simulink model "controlMCUSlugsMKII"  (Simulink 6.6)
settings: Solver=FixedStepDiscrete  StartTime=0.0  StopTime=10.0  FixedStep=0.01  RelTol=1e-3
InitFcn:
  | mcuInit
values from neighbouring files (symbols this model uses):
  T = 0.01    [initGPS.m]    (also in mcuInit.m)
undefined symbols (not defined in the file or in its folder): apSampleTime, bankCommandLimit, baseHeight, bda, bde, bdr, bdt, bICda, bICde, bICdr, bICdt, controlMCUInit, daLimit, deLimit, drLimit, dtLimit, getAccBias, getAccels, getAttitude, getMidLevelCommands, getPassValues, getPidIdx, getWP, getXYZ, gsRead, ISA_g, mda, mde, mdr, mdt, mICda, mICde, mICdr, mICdt, pitchCommandLimit, prepareTelemetry, protParseDecode, protParseDecodeGS, readIpc, send2GS, setCurrentCommands, setDiagnosticFloat, setDiagnosticShort, setNavLat, setNavLong, setNavNav, u1, u2, updateEuler, updateLoad, updatePQR, updatePWM, updatePWM2, y1
libraries: dsPICdrivers x82, simulink x43, SLUGS_Library x27, aerolibconvert2 x3, aerolibutil x3
(part 5 of 5)

== matlab function Trim Vals/Bufffer IC/Buffer IC Channel ==
  data: latest input inherited; history output inherited
function history = bufferICValues(latest)
% This block supports an embeddable subset of the MATLAB language.
% See the help menu for details. 

persistent oldValues;

if isempty(oldValues)
    oldValues = uint16([0 0 0 0 0 0 0]);
end

history = uint16([0 0 0 0 0 0 0]);

for i=7:-1:2
    oldValues(i) = oldValues(i-1);
	history(i) = oldValues(i-1);
end
	
oldValues(1) = latest;
history(1) = latest;

== matlab function Inner Loop/ Navigation/Navigation/Compute WP Index/Compute P/Compute T in Frenet/Normalize Vector/Norm/Subsystem3/Embedded MATLAB Function ==
  data: x input inherited; y input inherited; xDoty output inherited
function xDoty = myDot(x,y)
% This block supports an embeddable subset of the MATLAB language.
% See the help menu for details. 

xDoty = x(1)*y(1) + x(2)*y(2) + x(3)*y(3);

== matlab function Trim Vals/Bufffer IC/Buffer IC Channel1 ==
  data: latest input inherited; history output inherited
function history = bufferICValues(latest)
% This block supports an embeddable subset of the MATLAB language.
% See the help menu for details. 

persistent oldValues;

if isempty(oldValues)
    oldValues = uint16([0 0 0 0 0 0 0]);
end

history = uint16([0 0 0 0 0 0 0]);

for i=7:-1:2
    oldValues(i) = oldValues(i-1);
	history(i) = oldValues(i-1);
end
	
oldValues(1) = latest;
history(1) = latest;

== matlab function Inner Loop/ Navigation/Longitudinal Channel/Compute Airspeed/Subsystem1/negprotect ==
  data: val input inherited; zpVal output inherited
function zpVal = negProt(val)
% This block supports an embeddable subset of the MATLAB language.
% See the help menu for details. 

if val >= single(0.001)
    zpVal = val;
else
    zpVal = single(0.001);
end

== matlab function Inner Loop/ Navigation/Navigation/Compute WP Index/Compute P/Get Circles/Compute Circles ==
  data: sd input inherited; O output inherited; cd input inherited; WP1 input inherited; R input inherited; T1 input inherited; P output inherited; Pch output inherited; T2 input inherited; PchB output inherited
function [O,P,Pch, PchB] = getO(sd, cd, WP1, R, T1, T2)
    % This block supports an embeddable subset of the MATLAB language.
    % See the help menu for details.

    % rotate the vector delta degrees
    r_vec = zeros(3,1);
    r_vec(1) = -T1(1)*cd -T1(2)*sd;
    r_vec(2) = T1(1)*sd -T1(2)*cd;

    %compute M
    if localAbs(sd)>0.01
        M = localAbs(R/sd);
    else
        M = single(0);
    end

    %find the distance from WP
    P = M*cd;

    % find the center of the circle
    O = WP1 + r_vec.*M;

    % find the tangent points
    Pch = WP1-T1*P;
    PchB = WP1 + T2*P;
end

function absVal = localAbs(x)
    if x < 0
        absVal = single(-1*x);
    else
        absVal = single(x);
    end
end

== matlab function Inner Loop/ Navigation/Navigation/Compute WP Index/Compute P/Get Circles/Compute CCW Angle From 2 Vectors/Embedded MATLAB Function1 ==
  data: rawAngle input inherited; angle output inherited
function angle = mapToTwoPi(rawAngle)

 if(rawAngle < 0)
  angle = rawAngle + 2*pi;
 else
  angle = rawAngle;   
 end

== matlab function Inner Loop/ Navigation/Navigation/Compute WP Index/Embedded MATLAB Function ==
  data: wpStart input inherited; wpCount input inherited; wp0 output inherited; swIncrement input inherited; wp1 output inherited; wp2 output inherited; wpEnabl input inherited
function [wp0,wp1, wp2] = getNextWP(wpStart, wpCount, swIncrement, wpEnabl)

% Declare static variables
persistent fromWP;
persistent toWP;
persistent totoWP;

%initialize the static variables
if isempty(fromWP)
    fromWP = uint8(wpStart);
    toWP = uint8(fromWP+1);
    % check if there are more than 2 WPs
    if wpCount > toWP + 1
        totoWP = uint8(toWP+1);
    else
        totoWP = uint8(fromWP);
    end
end

%if WP Nav was just enabled
if wpEnabl == 1
    fromWP = uint8(0);
    toWP = uint8(1);
    totoWP = uint8(2);
end;

% if there is a change of wp
if swIncrement == 1
    fromWP = toWP;
    toWP = totoWP;
    totoWP = totoWP +1;
    if (totoWP>wpCount)
        totoWP = wpStart;
    end
end

wp0 = fromWP;
wp1 = toWP;
wp2 = totoWP;

== matlab function Inner Loop/ Navigation/Navigation/Compute WP Index/Embedded MATLAB Function1 ==
  data: swDistanceRdy input inherited; timeLimit input inherited; swIncrement output inherited
function swIncrement  = computeSwitch(swDistanceRdy, timeLimit)

% Declare static variables
persistent oldSw;
persistent internalTimer;

%initialize the static variables
if isempty(oldSw)
    oldSw = uint8(0);
    internalTimer = uint16(0);
    % check if there are more than 2 WPs
end 

swIncrement = 0;

%if we just had a flip
if swDistanceRdy == 1 && oldSw == 0
    % if enough time has passed that another switch is valid
    if internalTimer > timeLimit
        swIncrement = 1;
        internalTimer = uint16(0);
    end
end;

internalTimer = internalTimer +1;
oldSw = swDistanceRdy;

== matlab function Inner Loop/ Navigation/Longitudinal Channel/myMux Fun1 ==
  data: u1 input inherited; y output inherited; u2 input inherited
function y = myMux(u1, u2)
% This block supports an embeddable subset of the MATLAB language.
% See the help menu for details. 

y = [u1(1); u2(1)];

== matlab function Inner Loop/ Navigation/Navigation/Park, Deyst & How Lat Accel Cmd/myMux Fun2 ==
  data: u1 input inherited; y output inherited; u2 input inherited; u3 input inherited
function y = myMux(u1, u2, u3)
% This block supports an embeddable subset of the MATLAB language.
% See the help menu for details. 

y = [u1(1); u2(1); u3(1)];

== matlab function Inner Loop/ Navigation/Longitudinal Channel/0.5 sec  tau for Turns/Embedded MATLAB Function ==
  data: u input inherited; y output inherited; T input inherited; f input inherited
function y = fcn(u,T,f)
% This block supports an embeddable subset of the MATLAB language.
% See the help menu for details. 

persistent a
persistent b
persistent y_km1
persistent u_km1
if isempty(a)
    %tf = [T*omega/(2+T*omega) T*omega/(2+T*omega)],[1 (T*omega-2)/(T*omega+2)]
    %tf = [a a],[1 -b]
    omega = 2*pi*f;
    a=T*omega/(2+T*omega);
    b=-(T*omega-2)/(T*omega+2);
    y_km1=u;
    u_km1=u;
end

y = a*(u+u_km1)+b*y_km1;
y_km1=y;
u_km1=u;

== matlab function Inner Loop/ Navigation/Lateral Channel/Sideslip Compensation/Bank to Psi Dot/negprotect ==
  data: val input inherited; zpVal output inherited
function zpVal = negProt(val)
% This block supports an embeddable subset of the MATLAB language.
% See the help menu for details. 

if val >= single(0.001)
    zpVal = val;
else
    zpVal = single(0.001);
end

== matlab function Inner Loop/ Navigation/Navigation/Park, Deyst & How Lat Accel Cmd/Compute Eta/negprotect ==
  data: val input inherited; zpVal output inherited
function zpVal = negProt(val)
% This block supports an embeddable subset of the MATLAB language.
% See the help menu for details. 

if val >= single(0.001)
    zpVal = val;
else
    zpVal = single(0.001);
end

== matlab function Inner Loop/ Navigation/Navigation/Park, Deyst & How Lat Accel Cmd/GainSchedule L2 and Get Groundspeed/Norm /Square Vx and Vy Only. Vz is not considered CAREFUL/Embedded MATLAB Function ==
  data: x input inherited; y input inherited; xDoty output inherited
function xDoty = myDot(x,y)
% This block supports an embeddable subset of the MATLAB language.
% See the help menu for details. 

xDoty = x(1)*y(1) + x(2)*y(2);

== matlab function Inner Loop/ Navigation/Lateral Channel/myMux Fun1 ==
  data: u1 input inherited; y output inherited; u2 input inherited; u3 input inherited
function y = myMux(u1, u2, u3)
% This block supports an embeddable subset of the MATLAB language.
% See the help menu for details. 

y = [u1(1); u2(1); u3(1)];

== matlab function Inner Loop/ Navigation/Navigation/Compute WP Index/myMux Fun2 ==
  data: u1 input inherited; y output inherited; u2 input inherited; u3 input inherited; u4 input inherited
function y = myMux(u1, u2, u3, u4)
% This block supports an embeddable subset of the MATLAB language.
% See the help menu for details. 

y = [u1(1); u2(1); u3(1); u4(1)];

== matlab function Update PWM Commands and Send Telemetry/Generate PWM Signals Based on the Control Type/If  Control Type Is Wp Follow or Inner Cmds/myMux Fun1 ==
  data: u1 input inherited; y output inherited; u2 input inherited; u3 input inherited; u4 input inherited
function y = myMux(u1, u2, u3, u4 )
% This block supports an embeddable subset of the MATLAB language.
% See the help menu for details. 

y = [u1(1); u2(1); u3(1); u4(1)];

== matlab function Update PWM Commands and Send Telemetry/Generate PWM Signals Based on the Control Type/If  Control Type Is Passthrough/myMux Fun1 ==
  data: u1 input inherited; y output inherited; u2 input inherited; u3 input inherited; u4 input inherited
function y = myMux(u1, u2, u3, u4 )
% This block supports an embeddable subset of the MATLAB language.
% See the help menu for details. 

y = [u1(1); u2(1); u3(1); u4(1)];

== matlab function Update PWM Commands and Send Telemetry/Generate PWM Signals Based on the Control Type/If  Control Type Is Selective Passthrough/myMux Fun1 ==
  data: u1 input inherited; y output inherited; u2 input inherited; u3 input inherited; u4 input inherited
function y = myMux(u1, u2, u3, u4 )
% This block supports an embeddable subset of the MATLAB language.
% See the help menu for details. 

y = [u1(1); u2(1); u3(1); u4(1)];

== matlab function Update PWM Commands and Send Telemetry/myMux Fun1 ==
  data: u1 input inherited; y output inherited; u2 input inherited
function y = myMux(u1, u2)
% This block supports an embeddable subset of the MATLAB language.
% See the help menu for details. 

y = [u1(1:4); u2(1)];

== matlab function get Nav Vars/Embedded MATLAB Function ==
  data: u input inherited; y output inherited
function y = TwoPi(u)
% This block supports an embeddable subset of the MATLAB language.
% See the help menu for details. 

if ( u < 0 )
    y = u + 2*pi;
else
    y = u;
end

== matlab function Trim Vals/Bufffer IC/Buffer IC Channel2 ==
  data: latest input inherited; history output inherited
function history = bufferICValues(latest)
% This block supports an embeddable subset of the MATLAB language.
% See the help menu for details. 

persistent oldValues;

if isempty(oldValues)
    oldValues = uint16([0 0 0 0 0 0 0]);
end

history = uint16([0 0 0 0 0 0 0]);

for i=7:-1:2
    oldValues(i) = oldValues(i-1);
	history(i) = oldValues(i-1);
end
	
oldValues(1) = latest;
history(1) = latest;

== matlab function Trim Vals/Bufffer IC/Buffer IC Channel3 ==
  data: latest input inherited; history output inherited
function history = bufferICValues(latest)
% This block supports an embeddable subset of the MATLAB language.
% See the help menu for details. 

persistent oldValues;

if isempty(oldValues)
    oldValues = uint16([0 0 0 0 0 0 0]);
end

history = uint16([0 0 0 0 0 0 0]);

for i=7:-1:2
    oldValues(i) = oldValues(i-1);
	history(i) = oldValues(i-1);
end
	
oldValues(1) = latest;
history(1) = latest;

== matlab function Inner Loop/ Navigation/Navigation/myMux Fun3 ==
  data: u1 input inherited; y output inherited; u2 input inherited; u3 input inherited
function y = myMux(u1, u2, u3)
% This block supports an embeddable subset of the MATLAB language.
% See the help menu for details. 

y = [u1(1); u2(1); u3(1)];

== matlab function get Nav Vars/myMux Fun1 ==
  data: u1 input inherited; y output inherited; u2 input inherited; u3 input inherited
function y = myMux3(u1, u2, u3)
% This block supports an embeddable subset of the MATLAB language.
% See the help menu for details. 

y = [u1(1); u2(1); u3(1)];

== matlab function get Nav Vars/myMux Fun2 ==
  data: u1 input inherited; y output inherited; u2 input inherited
function y = myMux3(u1, u2)
% This block supports an embeddable subset of the MATLAB language.
% See the help menu for details. 

y = [u1(1:3); u2(1:3)];

== matlab function get Nav Vars/Euler Angles to Direction Cosine Matrix1/Create Transformation Matrix/myMux Fun1 ==
  data: u1 input inherited; y output inherited; u2 input inherited; u3 input inherited; u4 input inherited; u5 input inherited; u6 input inherited; u7 input inherited; u8 input inherited; u9 input inherited
function y = myMux3(u1, u2, u3, u4, u5, u6, u7, u8, u9)
% This block supports an embeddable subset of the MATLAB language.
% See the help menu for details. 

y = [u1(1); u2(1); u3(1);u4(1); u5(1); u6(1); u7(1); u8(1); u9(1)];

== matlab function get Nav Vars/Euler Angles to Direction Cosine Matrix2/Create Transformation Matrix/myMux Fun1 ==
  data: u1 input inherited; y output inherited; u2 input inherited; u3 input inherited; u4 input inherited; u5 input inherited; u6 input inherited; u7 input inherited; u8 input inherited; u9 input inherited
function y = myMux3(u1, u2, u3, u4, u5, u6, u7, u8, u9)
% This block supports an embeddable subset of the MATLAB language.
% See the help menu for details. 

y = [u1(1); u2(1); u3(1);u4(1); u5(1); u6(1); u7(1); u8(1); u9(1)];

== matlab function get Nav Vars/Euler Angles to Direction Cosine Matrix1/Subsystem5/myMux Fun1 ==
  data: u1 input inherited; y output inherited; u2 input inherited; u3 input inherited
function y = myMux3(u1, u2, u3)
% This block supports an embeddable subset of the MATLAB language.
% See the help menu for details. 

y = [u1(1); u2(1); u3(1)];

== matlab function get Nav Vars/Euler Angles to Direction Cosine Matrix1/Subsystem5/myMux Fun2 ==
  data: u1 input inherited; y output inherited; u2 input inherited; u3 input inherited
function y = myMux3(u1, u2, u3)
% This block supports an embeddable subset of the MATLAB language.
% See the help menu for details. 

y = [u1(1); u2(1); u3(1)];

== matlab function get Nav Vars/Euler Angles to Direction Cosine Matrix2/Subsystem5/myMux Fun1 ==
  data: u1 input inherited; y output inherited; u2 input inherited; u3 input inherited
function y = myMux3(u1, u2, u3)
% This block supports an embeddable subset of the MATLAB language.
% See the help menu for details. 

y = [u1(1); u2(1); u3(1)];

== matlab function get Nav Vars/Euler Angles to Direction Cosine Matrix2/Subsystem5/myMux Fun2 ==
  data: u1 input inherited; y output inherited; u2 input inherited; u3 input inherited
function y = myMux3(u1, u2, u3)
% This block supports an embeddable subset of the MATLAB language.
% See the help menu for details. 

y = [u1(1); u2(1); u3(1)];

== matlab function Inner Loop/ Navigation/Navigation/Park, Deyst & How Lat Accel Cmd/GainSchedule L2 and Get Groundspeed/negprotect1 ==
  data: val input inherited; zpVal output inherited
function zpVal = negProt(val)
% This block supports an embeddable subset of the MATLAB language.
% See the help menu for details. 

if val >= single(0.001)
    zpVal = val;
else
    zpVal = single(0.001);
end

== matlab function Inner Loop/ Navigation/Lateral Channel/0.5 sec  tau/Embedded MATLAB Function ==
  data: u input inherited; y output inherited; T input inherited; f input inherited
function y = fcn(u,T,f)
% This block supports an embeddable subset of the MATLAB language.
% See the help menu for details. 

persistent a
persistent b
persistent y_km1
persistent u_km1
if isempty(a)
    %tf = [T*omega/(2+T*omega) T*omega/(2+T*omega)],[1 (T*omega-2)/(T*omega+2)]
    %tf = [a a],[1 -b]
    omega = 2*pi*f;
    a=T*omega/(2+T*omega);
    b=-(T*omega-2)/(T*omega+2);
    y_km1=u;
    u_km1=u;
end

y = a*(u+u_km1)+b*y_km1;
y_km1=y;
u_km1=u;

== matlab function Inner Loop/ Navigation/Lateral Channel/Bank to Psi Dot/negprotect ==
  data: val input inherited; zpVal output inherited
function zpVal = negProt(val)
% This block supports an embeddable subset of the MATLAB language.
% See the help menu for details. 

if val >= single(0.1)
    zpVal = val;
else
    zpVal = single(0.001);
end

== matlab function Inner Loop/ Navigation/Navigation/Compute WP Index/Switch when in Line Segment/Compute Total Run/Compute Distance/Norm/Subsystem3/Embedded MATLAB Function ==
  data: x input inherited; y input inherited; xDoty output inherited
function xDoty = myDot(x,y)
% This block supports an embeddable subset of the MATLAB language.
% See the help menu for details. 

xDoty = x(1)*y(1) + x(2)*y(2) + x(3)*y(3);

== matlab function Inner Loop/ Navigation/Longitudinal Channel/5 sec tau for high speeds/Embedded MATLAB Function ==
  data: u input inherited; y output inherited; T input inherited; f input inherited
function y = fcn(u,T,f)
% This block supports an embeddable subset of the MATLAB language.
% See the help menu for details. 

persistent a
persistent b
persistent y_km1
persistent u_km1
if isempty(a)
    %tf = [T*omega/(2+T*omega) T*omega/(2+T*omega)],[1 (T*omega-2)/(T*omega+2)]
    %tf = [a a],[1 -b]
    omega = 2*pi*f;
    a=T*omega/(2+T*omega);
    b=-(T*omega-2)/(T*omega+2);
    y_km1=u;
    u_km1=u;
end

y = a*(u+u_km1)+b*y_km1;
y_km1=y;
u_km1=u;

== matlab function Inner Loop/ Navigation/Longitudinal Channel/0.3 sec  tau for low speeds/Embedded MATLAB Function ==
  data: u input inherited; y output inherited; T input inherited; f input inherited
function y = fcn(u,T,f)
% This block supports an embeddable subset of the MATLAB language.
% See the help menu for details. 

persistent a
persistent b
persistent y_km1
persistent u_km1
if isempty(a)
    %tf = [T*omega/(2+T*omega) T*omega/(2+T*omega)],[1 (T*omega-2)/(T*omega+2)]
    %tf = [a a],[1 -b]
    omega = 2*pi*f;
    a=T*omega/(2+T*omega);
    b=-(T*omega-2)/(T*omega+2);
    y_km1=u;
    u_km1=u;
end

y = a*(u+u_km1)+b*y_km1;
y_km1=y;
u_km1=u;
